simulink model "activeCellBalancing"  (R2023a)
settings: Solver=VariableStepAuto  StartTime=0.0  StopTime=3600  RelTol=1e-3
libraries: spsVoltageMeasurementLib x4, spsDiodeLib x2, spsSeriesRLCBranchLib x2, spsGroundLib x1, spsLinearTransformerLib x1, spsMosfetLib x1, sps_lib x1
settings Model: Creator=DELL  LastModifiedBy=DELL

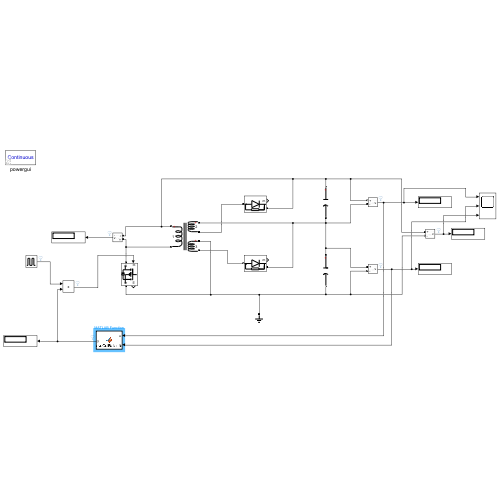
[thumbnail: Simulink's stored preview of the top-level diagram]
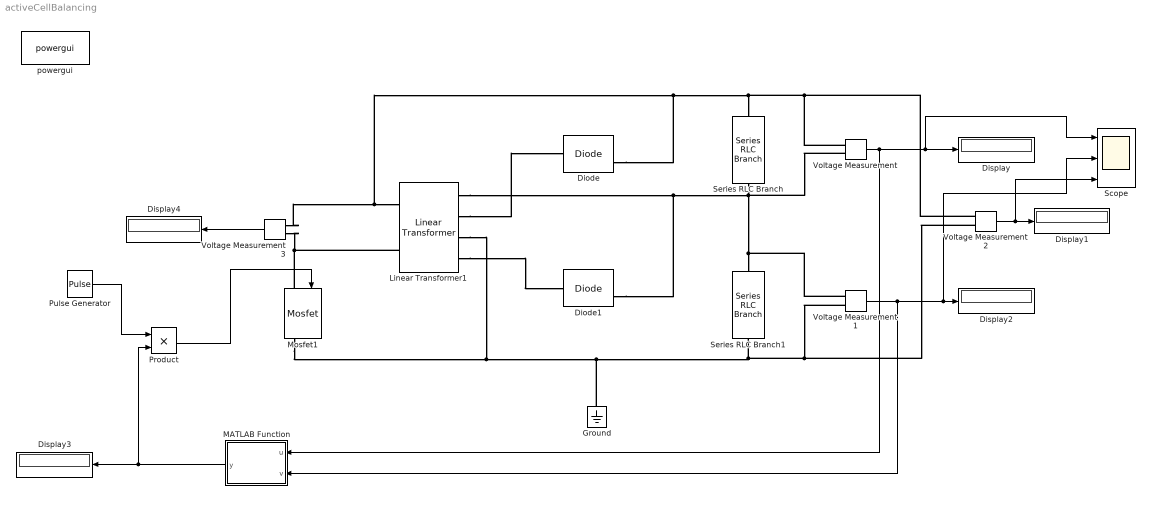
== system activeCellBalancing ==
  Diode : spsDiodeLib/Diode  Ron=0.001  Lon=0  Vf=0.8  IC=0  UseSnubber=0  Rs=1500  Cs=288e-7  Measurements=on
  Diode1 : spsDiodeLib/Diode  Ron=0.001  Lon=0  Vf=0.8  IC=0  UseSnubber=0  Rs=1500  Cs=288e-7  Measurements=on
  Display{,1..4} (5 alike) : Display
  Ground : spsGroundLib/Ground  LConnTagsString=a
  Linear Transformer1 : spsLinearTransformerLib/Linear Transformer  UNITS=SI  NominalPower=[ 100 55000 ]  winding1=[10 0.02 45e-6]  winding2=[5 0.02 288e-6]  ThreeWindings=on  winding3=[5 0.02 288e-6]  RmLm=[1.0804e+06 2866]  Measurements=None  DataType=on
  MATLAB Function : MATLAB Function  TreatAsAtomicUnit=on
  Mosfet1 : spsMosfetLib/Mosfet  Ron=1.5  Lon=0  Rd=2  Vfd=0  IC=0  Rs=1500  Cs=288e-7  Measurements=on
  Product : Product
  Pulse Generator : DiscretePulseGenerator  PulseType=Time based  Period=10  PulseWidth=5
  Scope : Scope  NumInputPorts=3
  Series RLC Branch : spsSeriesRLCBranchLib/Series RLC Branch  LConnTagsString=__new0  RConnTagsString=__new0  BranchType=C  Resistance=1  Inductance=1e-3  SetiL0=off  InitialCurrent=0  Capacitance=5  Setx0=on  InitialVoltage=2  Measurements=None
  Series RLC Branch1 : spsSeriesRLCBranchLib/Series RLC Branch  LConnTagsString=__new0  RConnTagsString=__new0  BranchType=C  Resistance=1  Inductance=1e-3  SetiL0=off  InitialCurrent=0  Capacitance=5  Setx0=on  InitialVoltage=4  Measurements=None
  Voltage Measurement{,1..3} (4 alike) : spsVoltageMeasurementLib/Voltage Measurement  PhasorSimulation=off  OutputType=Complex  PSBequivalent=0
  powergui : sps_lib/powergui  Priority=1  SimulationMode=Continuous  SampleTime=50e-6  frequency=60  Iterations=50  frequencyindice=0  Pbase=100e6  ErrMax=1e-4  UnitsV=kV  UnitsW=MW  buscounter=0  FunctionMessages=off  echomessages=off  EnableUseOfTLC=off  CurrentSourceSwitches=off  DisableSnubberDevices=off  DisableRonSwitches=off  DisableVfSwitches=off  DisplayEquations=off  AutomaticDiscreteSolvers=off  SolverType=Tustin/Backward Euler (TBE)  Interpol=off  ExternalGateDelay=off  methode=off  Ts=100  x0status=blocks  SPID=on  SwTol=0  HookPort=off  NonlinearTolerance=1e-4  nMaxIteration=100  ContinueOnMaxIteration=off  RestoreLinks=warning  ResistiveCurrentMeasurement=off  Frange=[0:2:500]  Ylog=off  Xlog=on  ShowGrid=off  save=off  variable=ZData  structure=0  ZoomFFT=off  StartTime=0.0  cycles=1  DisplayStyle=1  fundamental=60  FreqAxis=off  MaxFrequency=1000  frequencyindicesteady=1  RmsSteady=1  display=off
  wires:
  Pulse Generator/1 -> Product/1
  Product/1 -> Mosfet1/1
  MATLAB Function/1(y) -> Product/2, Display3/1
  Voltage Measurement/1 -> MATLAB Function/1(u), Scope/1, Display/1
  Voltage Measurement1/1 -> MATLAB Function/2(v), Scope/2, Display2/1
  Voltage Measurement2/1 -> Scope/3, Display1/1
  Voltage Measurement3/1 -> Display4/1
  connections:
  Linear Transformer1/RConn2 -- Diode/LConn1
  Diode/RConn1 -- Linear Transformer1/LConn1 -- Voltage Measurement3/LConn2 -- Series RLC Branch/LConn1 -- Voltage Measurement/LConn1 -- Voltage Measurement2/LConn1
  Linear Transformer1/RConn4 -- Diode1/LConn1
  Mosfet1/RConn1 -- Linear Transformer1/RConn3 -- Ground/LConn1 -- Voltage Measurement1/LConn2 -- Voltage Measurement2/LConn2 -- Series RLC Branch1/RConn1
  Voltage Measurement3/LConn1 -- Mosfet1/LConn1 -- Linear Transformer1/LConn2
  Series RLC Branch/RConn1 -- Voltage Measurement/LConn2 -- Linear Transformer1/RConn1 -- Diode1/RConn1 -- Voltage Measurement1/LConn1 -- Series RLC Branch1/LConn1

== matlab function activeCellBalancing/MATLAB Function ==
  data: u input; y output; v input
function y = fcn(u, v)
    if u == v
        y = 0;
    else
        y = 1;
    end
end
